simulink model "Fig424"  (R2014b)
settings: Solver=ode3  StartTime=0.0  StopTime=.005  FixedStep=1.5625e-6  RelTol=1e-3
libraries: commsrccod2 x2, dspquant2 x2, commutil2 x1, dspsigops x1, dsparch4 x1
settings Model: DataTypeOverride=Double  MinMaxOverflowLogging=ForceOff  Creator=Dennis Silage  LastModifiedBy=Silage
settings DataIOCC: SignalLoggingSaveFormat=ModelDataLogs
settings OptimizationCC: ExpressionDepthLimit=2147483647  InitFltsAndDblsToZero=on
settings DebuggingCC: UnderspecifiedInitializationDetection=Classic  MergeDetectMultiDrivingBlocksExec=none  FcnCallInpInsideContextMsg=UseLocalSettings  UnconnectedOutputMsg=none  StateNameClashWarn=warning
settings GRTTargetCC: CombineOutputUpdateFcns=off  GRTInterface=on

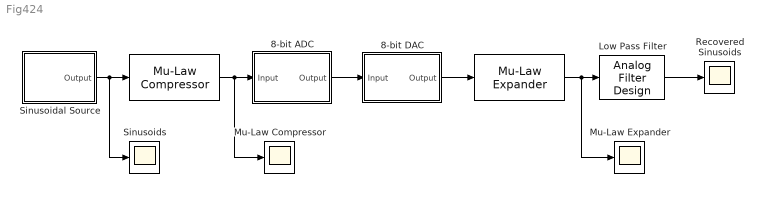
== system Fig424 ==
  "   " : commsrccod2/Mu-Law Compressor  mu=255  V=1.28
  "    " : commsrccod2/Mu-Law Expander  mu=255  V=1.28
  8-bit ADC : Subsystem
  8-bit DAC : Subsystem
  Low Pass Filter : dsparch4/Analog Filter Design  method=Butterworth  filttype=Lowpass  N=9  Wlo=7500*pi  Whi=80  Rp=2  Rs=40
  Mu-Law Compressor : Scope
      settings: YMin=-1.5  YMax=1.5
  Mu-Law Expander : Scope
      settings: YMin=-1.5  YMax=1.5
  Recovered Sinusoids : Scope
      settings: YMin=-1.5  YMax=1.5  SaveName=ScopeData4
  Sinusoidal Source : Subsystem
  Sinusoids : Scope
      settings: YMin=-1.5  YMax=1.5  SaveName=ScopeData2
  wires:
  Sinusoidal Source/1(Output) -> "   "/1, Sinusoids/1
  8-bit ADC/1(Output) -> 8-bit DAC/1(Input)
  "   "/1 -> Mu-Law Compressor/1, 8-bit ADC/1(Input)
  8-bit DAC/1(Output) -> "    "/1
  "    "/1 -> Mu-Law Expander/1, Low Pass Filter/1
  Low Pass Filter/1 -> Recovered Sinusoids/1

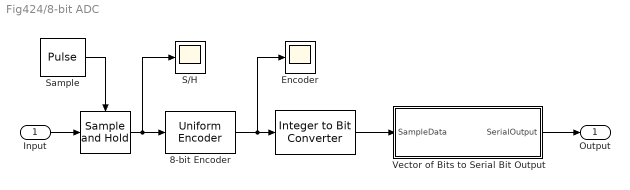
== system Fig424/8-bit ADC ==
  Input : Inport
  " " : commutil2/Integer to Bit Converter  nbits=8  signedInputValues=Unsigned  bitOrder=LSB first  outDtype=uint8
  "   " : dspsigops/Sample and Hold  trig=Rising edge  initCond=0  latchinput=off
  8-bit Encoder : dspquant2/Uniform Encoder  peak=1.28  bits=8  otype=Unsigned integer
  Encoder : Scope
      settings: YMin=-10  YMax=275  SaveName=ScopeData3
  S/H : Scope
      settings: YMin=-1.5  YMax=1.5  SaveName=ScopeData6
  Sample : DiscretePulseGenerator  Period=80  PulseWidth=8  SampleTime=1.5625e-6
  Vector of Bits to Serial Bit Output : MATLAB Function  TreatAsAtomicUnit=on
  Output : Outport
  wires:
  Sample/1 -> "   "/Trigger
  "   "/1 -> S/H/1, 8-bit Encoder/1
  Input/1 -> "   "/1
  Vector of Bits to Serial Bit Output/1(SerialOutput) -> Output/1
  8-bit Encoder/1 -> Encoder/1, " "/1
  " "/1 -> Vector of Bits to Serial Bit Output/1(SampleData)

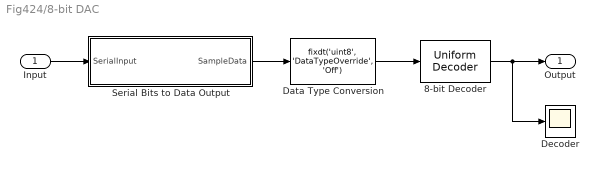
== system Fig424/8-bit DAC ==
  Input : Inport
  8-bit Decoder : dspquant2/Uniform Decoder  peak=1.28  bits=8  overflowMode=Saturate  otype=Double
  Data Type Conversion : DataTypeConversion  OutDataTypeStr=fixdt('uint8', 'DataTypeOverride', 'Off')  LockScale=on
  Decoder : Scope
      settings: YMin=-1.5  YMax=1.5  SaveName=ScopeData5
  Serial Bits to Data Output : MATLAB Function  TreatAsAtomicUnit=on
  Output : Outport
  wires:
  Input/1 -> Serial Bits to Data Output/1(SerialInput)
  8-bit Decoder/1 -> Decoder/1, Output/1
  Serial Bits to Data Output/1(SampleData) -> Data Type Conversion/1
  Data Type Conversion/1 -> 8-bit Decoder/1

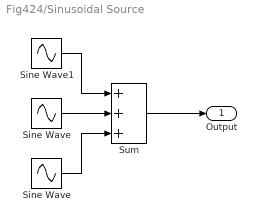
== system Fig424/Sinusoidal Source ==
  " Sine Wave " : Sin  Amplitude=0.2  Frequency=5000*pi  SampleTime=1.5625e-6
  "Sine Wave " : Sin  Amplitude=0.5  Frequency=3000*pi  SampleTime=1.5625e-6
  Sine Wave1 : Sin  Frequency=1000*pi  SampleTime=1.5625e-6
  Sum : Sum  Inputs=+++
  Output : Outport
  wires:
  "Sine Wave "/1 -> Sum/2
  " Sine Wave "/1 -> Sum/3
  Sine Wave1/1 -> Sum/1
  Sum/1 -> Output/1

== matlab function Fig424/8-bit DAC/Serial Bits to Data Output ==
  data: SerialInput input; SampleData output
function SampleData = fcn(SerialInput)
%#codegen

persistent SmpDat SmpNum SmpDatOld

if isempty(SmpNum)
    SmpNum = 0;
    SmpDat = 0;
    SmpDatOld = 0;
    SampleData = 0; %#ok<NASGU>
end

SmpNum = SmpNum + 1;
if (SmpNum == 9)
    SmpNum = 1;
    SampleData = SmpDat;
    SmpDatOld = SmpDat;
    SmpDat = SerialInput;
else
    SampleData = SmpDatOld;
    SmpDat = SmpDat + SerialInput*2^(SmpNum-1);
end

end

== matlab function Fig424/8-bit ADC/Vector of Bits to Serial Bit Output ==
  data: SampleData input; SerialOutput output
function SerialOutput = fcn(SampleData)
%#codegen
persistent SmpNum

if isempty(SmpNum)
    SmpNum = 1;
end

SerialOutput = SampleData(SmpNum);
SmpNum = SmpNum + 1;
if (SmpNum == 9)
    SmpNum = 1;
end

end
